simulink model "BodeSimulacion1_2"  (R2024a)
settings: Solver=ode45  StartTime=0.0  StopTime=5  MaxStep=0.00001  RelTol=1e-3  EnableMultiTasking=on
InitFcn:
  | BodeSimParametros
values from neighbouring files (symbols this model uses):
  T = 0.2    [BodeSimParametros.m]
  wi = 2*pi*f    (= 62.8318530718)    [BodeSimParametros.m]
  wn = 2*pi*f2    (= 31415.9265359)    [BodeSimParametros.m]    (also in BodeTerminosSimples.m = 10)
  wn2 = 2*pi*10    (= 62.8318530718)    [BodeSimParametros.m]
  wr = wn2*sqrt(1-2*xi2^2)    [BodeSimParametros.m]    (also in BodeTerminosSimples.m = wn*sqrt(1-2*xi^2))
  wz = 2*pi*28000    (= 175929.188601)    [BodeSimParametros.m]
  xi = 1/sqrt(2)    [BodeSimParametros.m]    (also in BodeTerminosSimples.m = 0.5)
  xi2 = 0.05    [BodeSimParametros.m]
settings Model: Creator=Gera  LastModifiedBy=david
settings SolverCC: AlgebraicLoopSolver=TrustRegion
settings DataIOCC: LimitDataPoints=on  SaveFormat=Array  SignalLoggingSaveFormat=ModelDataLogs  ReturnWorkspaceOutputs=off
settings OptimizationCC: ExpressionDepthLimit=2147483647  InitFltsAndDblsToZero=on  LifeSpan=inf
settings DebuggingCC: UnderspecifiedInitializationDetection=Classic  MergeDetectMultiDrivingBlocksExec=none  SolverPrmCheckMsg=warning  FcnCallInpInsideContextMsg=warning  UnconnectedInputMsg=warning  UnconnectedOutputMsg=warning  UnconnectedLineMsg=warning  StateNameClashWarn=warning  SFUnexpectedBacktrackingDiag=warning  SFNoUnconditionalDefaultTransitionDiag=warning  ArithmeticOperatorsInVariantConditions=warning
settings HardwareCC: ProdBitPerPointer=32  ProdBitPerSizeT=32  ProdBitPerPtrDiffT=32  ProdLargestAtomicFloat=None  ProdIntDivRoundTo=Undefined  ProdEndianess=Unspecified  ProdWordSize=32  ProdHWDeviceType=32-bit Generic
settings ModelReferenceCC: EnableRefExpFcnMdlSchedulingChecks=on  PropagateSignalLabelsOutOfModel=off
settings SFSimCC: SimUseLocalCustomCode=off  CustomCodeUndefinedFunction=UseInterfaceOnly
settings RTWCC: RTWUseLocalCustomCode=off  GPUComputeCapability=3.5  DLArmComputeVersion=19.05
settings CodeAppCC: StateflowObjectComments=on
settings GRTTargetCC: TargetLangStandard=C89/C90 (ANSI)  CombineOutputUpdateFcns=off  GRTInterface=on
settings ConfigComp: CovMetricSettings=dw  CovSaveCumulativeToWorkspaceVar=on  CovSaveSingleToWorkspaceVar=on  CovExternalEMLEnable=off  CovSFcnEnable=off

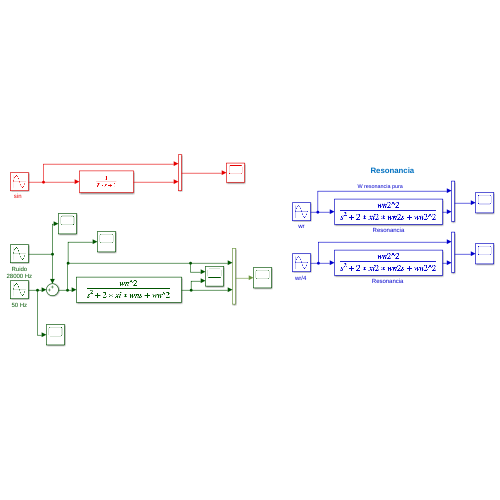
[thumbnail: Simulink's stored preview of the top-level diagram]
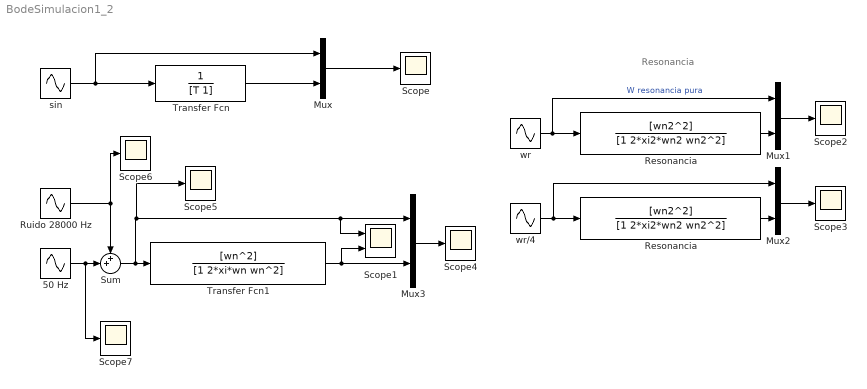
== system BodeSimulacion1_2 ==
  note: Resonancia
  50 Hz : Sin  Frequency=wi  SampleTime=0
  Mux{,1..3} (4 alike) : Mux  Inputs=2
  Resonancia : TransferFcn  Numerator=[wn2^2]  Denominator=[1 2*xi2*wn2 wn2^2]
  "Resonancia " : TransferFcn  Numerator=[wn2^2]  Denominator=[1 2*xi2*wn2 wn2^2]
  Ruido 28000 Hz : Sin  Amplitude=0.1  Frequency=wz  SampleTime=0
  Scope{,2..7} (7 alike) : Scope
  Scope1 : Scope  NumInputPorts=2
  Sum : Sum  Inputs=++|
  Transfer Fcn : TransferFcn  Denominator=[T 1]
  Transfer Fcn1 : TransferFcn  Numerator=[wn^2]  Denominator=[1 2*xi*wn wn^2]
  "sin  " : Sin  Frequency=wi  SampleTime=0
  wr : Sin  Amplitude=10  Frequency=wr  SampleTime=0
  "wr/4 " : Sin  Amplitude=10  Frequency=wr/4  SampleTime=0
  wires:
  "sin  "/1 -> Transfer Fcn/1, Mux/1
  Transfer Fcn/1 -> Mux/2
  Mux/1 -> Scope/1
  Transfer Fcn1/1 -> Mux3/2, Scope1/2
  50 Hz/1 -> Scope7/1, Sum/2
  Sum/1 -> Transfer Fcn1/1, Scope5/1, Mux3/1, Scope1/1
  Ruido 28000 Hz/1 -> Scope6/1, Sum/1
  wr/1 -> Resonancia/1, Mux1/1  "W resonancia pura"
  Resonancia/1 -> Mux1/2
  Mux1/1 -> Scope2/1
  "wr/4 "/1 -> "Resonancia "/1, Mux2/1
  Mux2/1 -> Scope3/1
  Mux3/1 -> Scope4/1
  "Resonancia "/1 -> Mux2/2
